simulink model "lorenz1"  (R2013a)
settings: Solver=ode4  StartTime=0.0  StopTime=5  FixedStep=0.001  RelTol=1e-6  AbsTol=1e-9
values from neighbouring files (symbols this model uses):
  k1 = (1-k1)/(1-0.4)    [cpso_pid1.m]    (also in loren2.m = x(i,1))
  k2 = (1-k2)/(1-0.4)    [cpso_pid1.m]    (also in loren2.m = x(i,2))
  k3 = (1-k3)/(1-0.4)    [cpso_pid1.m]    (also in loren2.m = x(i,3))
settings Model: Creator=Administrator  LastModifiedBy=sjp
settings SolverCC: ZeroCrossControl=DisableAll

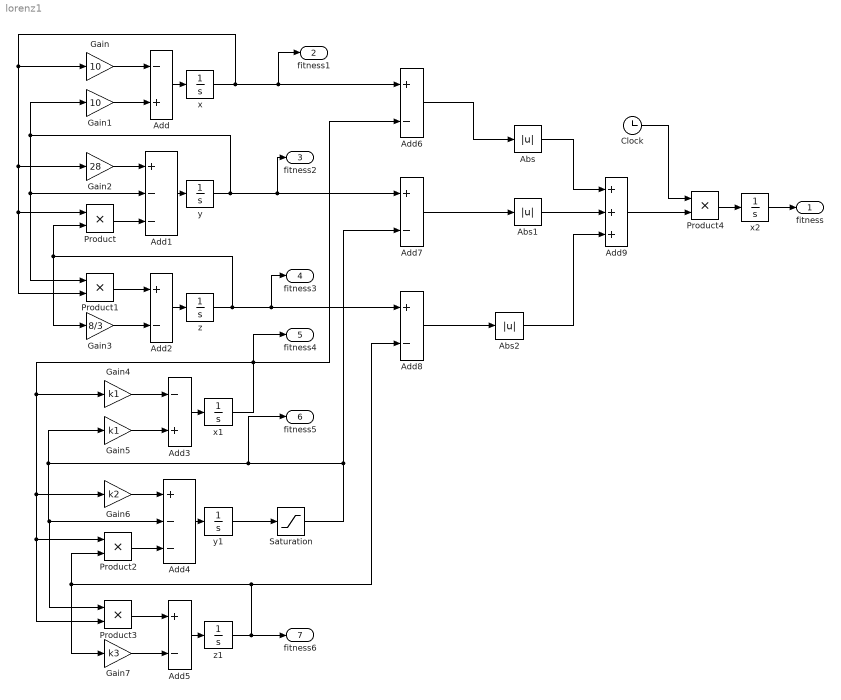
== system lorenz1 ==
  Abs : Abs
  Abs1 : Abs
  Abs2 : Abs
  Add : Sum  Inputs=-+
  Add1 : Sum  Inputs=+--
  Add{2,5..8} (5 alike) : Sum  Inputs=+-
  Add3 : Sum  Inputs=-+
  Add4 : Sum  Inputs=+--
  Add9 : Sum  Inputs=+++
  Clock : Clock
  Gain : Gain  Gain=10
  Gain1 : Gain  Gain=10
  Gain2 : Gain  Gain=28
  Gain3 : Gain  Gain=8/3
  Gain4 : Gain  Gain=k1
  Gain5 : Gain  Gain=k1
  Gain6 : Gain  Gain=k2
  Gain7 : Gain  Gain=k3
  Product{,1..4} (5 alike) : Product
  Saturation : Saturate  UpperLimit=80  LowerLimit=-80
  x : Integrator  InitialCondition=0.02
  x1 : Integrator  InitialCondition=0.02
  x2 : Integrator
  y : Integrator  InitialCondition=0.01
  y1 : Integrator  InitialCondition=0.01
  z : Integrator  InitialCondition=0.03
  z1 : Integrator  InitialCondition=0.03
  fitness : Outport
  fitness1 : Outport  Port=2
  fitness2 : Outport  Port=3
  fitness3 : Outport  Port=4
  fitness4 : Outport  Port=5
  fitness5 : Outport  Port=6
  fitness6 : Outport  Port=7
  wires:
  Add/1 -> x/1
  Add1/1 -> y/1
  Add2/1 -> z/1
  Gain/1 -> Add/1
  Gain1/1 -> Add/2
  Gain2/1 -> Add1/1
  Product/1 -> Add1/3
  x/1 -> fitness1/1, Add6/1, Product1/2, Product/1, Gain2/1, Gain/1
  y/1 -> fitness2/1, Add7/1, Product1/1, Add1/2, Gain1/1
  Gain3/1 -> Add2/2
  Product1/1 -> Add2/1
  z/1 -> Product/2, Gain3/1, fitness3/1, Add8/1
  Add3/1 -> x1/1
  Add4/1 -> y1/1
  Add5/1 -> z1/1
  Gain4/1 -> Add3/1
  Gain5/1 -> Add3/2
  Gain6/1 -> Add4/1
  Product2/1 -> Add4/3
  x1/1 -> fitness4/1, Add6/2, Product3/2, Product2/1, Gain6/1, Gain4/1
  Gain7/1 -> Add5/2
  Product3/1 -> Add5/1
  z1/1 -> Add8/2, Product2/2, Gain7/1, fitness6/1
  Add6/1 -> Abs/1
  Add7/1 -> Abs1/1
  Add8/1 -> Abs2/1
  Abs/1 -> Add9/1
  Abs1/1 -> Add9/2
  Abs2/1 -> Add9/3
  x2/1 -> fitness/1
  Clock/1 -> Product4/1
  Add9/1 -> Product4/2
  Product4/1 -> x2/1
  y1/1 -> Saturation/1
  Saturation/1 -> fitness5/1, Product3/1, Add4/2, Gain5/1, Add7/2
